simulink model "Microgrid_transition_model_FORFIG"  (R2020a)
settings: Solver=VariableStepAuto  StartTime=0.0  StopTime=16  MaxStep=1e-4  RelTol=1e-3
PreLoadFcn:
  | %run('FC_microgrid_param.m')
  | %load('gen_grid_init.mat')
InitFcn:
  | %load myisoModel_init;
  | run('FC_microgrid_param.m')
  | tic
  | run('CARTinitFcn.m')
  | %caseNo = 2;
  | 
  | %if (caseNo == 1)
  | %set_param(['Isolated_grid_paper_model_022521/SignalGen'], 'ActiveScenario', 'PStep222kW');
  | %else
  | %set_param(['Isolated_grid_paper_model_022521/SignalGen'], 'ActiveScenario', 'QStep222kVAr');
  | 
  | %end;
StopFcn:
  | toc
undefined symbols (not defined in the file): breakpoints1, breakpoints2, cp_table_data, ctrl, D1, Delta, DiscIntNeverNeededParam, DT, FC_BESS, find_system, gcbh, libFC_BESS, LowerLimit, magnitude, oversize, pq_ts, sps_rtmsupport, timer, Ts, ts, Ts_APC, Ts_Control, Ts_Power, UpperLimit
libraries: powerlib x130, powerlib_meascontrol x104, simulink x65, powerlib_extras x40, simulink_extras x16, eePowerMeasurement x9, sps_avr x7, pi_ctrl x4, spsDieselMotorModel x3, SignalEditorBlockLib x2, libLgBattery x1, libFC_PV x1
(part 5 of 13)

== system Microgrid_transition_model_FORFIG/Grid Feeder Protective Relay/RMS_Calculator2 ==
  note: % Copyright (c) 2016 Massachusetts Institute of Technology
      | % Permission is hereby granted, free of charge, to any person obtaining a copy of this
      | % software and associated documentation files (the "Software"), to deal in the Software
      | % without restriction, including without limitation the rights to use, copy, modify,
      | % merge, publish, distribute, sublicense, and/or sell copies of the Software, and to
      | % permit persons to whom the Software is furnished to do so, subject to the following
      | % conditions:
      | %
      | %
      | % The above copyright notice and this permission notice shall be included in
      | % all copies or substantial portions of the Software.
      | %
      | % THE SOFTWARE IS PROVIDED "AS IS", WITHOUT WARRANTY OF ANY KIND, EXPRESS OR IMPLIED,
      | % INCLUDING BUT NOT LIMITED TO THE WARRANTIES OF MERCHANTABILITY, FITNESS FOR A
      | % PARTICULAR PURPOSE AND NONINFRINGEMENT. IN NO EVENT SHALL THE AUTHORS OR COPYRIGHT
      | % HOLDERS BE LIABLE FOR ANY CLAIM, DAMAGES OR OTHER LIABILITY, WHETHER IN AN ACTION
      | % OF CONTRACT, TORT OR OTHERWISE, ARISING FROM, OUT OF OR IN CONNECTION WITH THE
      | % SOFTWARE OR THE USE OR OTHER DEALINGS IN THE SOFTWARE.
      | %
      | %
      | %%
  s : Inport
  Abs : Abs
  Discrete Mean value6 : powerlib_extras/Discrete Measurements/Discrete  Mean value  Freq=60  Vinit=0  Ts=Ts
      settings: SourceProductBaseCode=PS
  Product3 : Product  RndMeth=Zero
  Signed Sqrt : Sqrt  SaturateOnIntegerOverflow=on
  RMS : Outport
  wires:
  Signed Sqrt/1 -> RMS/1
  Discrete Mean value6/1 -> Abs/1
  s/1 -> Product3/2, Product3/1
  Product3/1 -> Discrete Mean value6/1
  Abs/1 -> Signed Sqrt/1

== system Microgrid_transition_model_FORFIG/Grid Feeder Protective Relay1/CS Modified PLL ==
  note: SPS Discrete 3-phase PLL
  note: Pierre Giroux, Gilbert Sybille
      | Power System Laboratory, IREQ
      | Hydro-Quebec
      | (August 2007)
  Vabc(pu) : Inport  PortDimensions=3
  2nd-Order Filter : powerlib_extras/Discrete  Control Blocks/Discrete  2nd-Order Filter  FilterType=Lowpass  Fo=25  Zeta=0.707  Ts=Ts  Initialize=on  Vac_Init=[0 0 Finit]  Vdc_Init=Finit  PlotResponse=off  param1=[1 500 0.1]
      settings: SourceProductBaseCode=PS
  Controller : Subsystem  mask(Discrete PID Controller){Kp=Kp, Ki=Ki, Kd=Kd, Par_Limits=[Flim(2) Flim(1)]*2*pi, Init=2*pi*Finit, Ts=Ts}
      mask prompts: Kp "Proportional gain (Kp):"; Ki "Integral gain (Ki):"; Kd "Derivative gain (Kd):"; Par_Limits "Output limits: [ Upper   Lower ]"; Init "Output initial value:"; Ts "Sample time:"
      mask help: This block implements a discrete PID controller.
      mask init:
      | UpperLimit=Par_Limits(1);
      | LowerLimit=Par_Limits(2);
      | power_initmask();
      settings: OpenFcn=power_openblockproxy();
      mask Display: disp('PID');
  Discrete Rate Limiter : powerlib_extras/Discrete  Control Blocks/Discrete Rate Limiter  R=12  F=-12  Vinit=Finit  Ts=Ts
      settings: SourceProductBaseCode=PS
  Discrete Mean value : powerlib_extras/Discrete Measurements/Discrete  Mean value  Freq=60  Vinit=0  Ts=Ts
      settings: SourceProductBaseCode=PS
  Gain10 : Gain  Gain=1/2/pi  SaturateOnIntegerOverflow=on  OutDataTypeStr=Inherit: Same as input  ParamDataTypeStr=Inherit: Same as input
  Mux2 : Mux  Inputs=2
  Selector : Selector  InputPortWidth=3  IndexOptions=Index vector (dialog)  Indices=2  OutputSizes=1
  Trigonometric Function : Trigonometry
  Trigonometric Function2 : Trigonometry  Operator=cos
  Unit Delay : UnitDelay  InitialCondition=Finit  SampleTime=Ts  HasFrameUpgradeWarning=on
  VCO : Subsystem
  abc_to_dq0 Transformation : powerlib_extras/Measurements/abc_to_dq0 Transformation
      settings: SourceProductBaseCode=PS
  Freq : Outport
  wt : Outport  Port=2
  Sin_Cos : Outport  Port=3
  wires:
  Discrete Mean value/1 -> Controller/1(Error)
  Controller/1(Out) -> VCO/1(w), Gain10/1  "W"
  Vabc(pu)/1 -> abc_to_dq0 Transformation/1
  abc_to_dq0 Transformation/1 -> Selector/1
  VCO/1(theta) -> Trigonometric Function/1, Trigonometric Function2/1, wt/1
  Trigonometric Function/1 -> Mux2/1
  Trigonometric Function2/1 -> Mux2/2
  Mux2/1 -> abc_to_dq0 Transformation/2, Sin_Cos/1
  Gain10/1 -> Discrete Rate Limiter/1
  Discrete Rate Limiter/1 -> 2nd-Order Filter/1
  Unit Delay/1 -> Freq/1
  2nd-Order Filter/1 -> Unit Delay/1
  Selector/1 -> Discrete Mean value/1  "Vq"

== system Microgrid_transition_model_FORFIG/Grid Feeder Protective Relay1/CS Modified PLL1 ==
  note: SPS Discrete 3-phase PLL
  note: Pierre Giroux, Gilbert Sybille
      | Power System Laboratory, IREQ
      | Hydro-Quebec
      | (August 2007)
  Vabc(pu) : Inport  PortDimensions=3
  2nd-Order Filter : powerlib_extras/Discrete  Control Blocks/Discrete  2nd-Order Filter  FilterType=Lowpass  Fo=25  Zeta=0.707  Ts=Ts  Initialize=on  Vac_Init=[0 0 Finit]  Vdc_Init=Finit  PlotResponse=off  param1=[1 500 0.1]
      settings: SourceProductBaseCode=PS
  Controller : Subsystem  mask(Discrete PID Controller){Kp=Kp, Ki=Ki, Kd=Kd, Par_Limits=[Flim(2) Flim(1)]*2*pi, Init=2*pi*Finit, Ts=Ts}
      mask prompts: Kp "Proportional gain (Kp):"; Ki "Integral gain (Ki):"; Kd "Derivative gain (Kd):"; Par_Limits "Output limits: [ Upper   Lower ]"; Init "Output initial value:"; Ts "Sample time:"
      mask help: This block implements a discrete PID controller.
      mask init:
      | UpperLimit=Par_Limits(1);
      | LowerLimit=Par_Limits(2);
      | power_initmask();
      settings: OpenFcn=power_openblockproxy();
      mask Display: disp('PID');
  Discrete Rate Limiter : powerlib_extras/Discrete  Control Blocks/Discrete Rate Limiter  R=12  F=-12  Vinit=Finit  Ts=Ts
      settings: SourceProductBaseCode=PS
  Discrete Mean value : powerlib_extras/Discrete Measurements/Discrete  Mean value  Freq=60  Vinit=0  Ts=Ts
      settings: SourceProductBaseCode=PS
  Gain10 : Gain  Gain=1/2/pi  SaturateOnIntegerOverflow=on  OutDataTypeStr=Inherit: Same as input  ParamDataTypeStr=Inherit: Same as input
  Mux2 : Mux  Inputs=2
  Selector : Selector  InputPortWidth=3  IndexOptions=Index vector (dialog)  Indices=2  OutputSizes=1
  Trigonometric Function : Trigonometry
  Trigonometric Function2 : Trigonometry  Operator=cos
  Unit Delay : UnitDelay  InitialCondition=Finit  SampleTime=Ts  HasFrameUpgradeWarning=on
  VCO : Subsystem
  abc_to_dq0 Transformation : powerlib_extras/Measurements/abc_to_dq0 Transformation
      settings: SourceProductBaseCode=PS
  Freq : Outport
  wt : Outport  Port=2
  Sin_Cos : Outport  Port=3
  wires:
  Discrete Mean value/1 -> Controller/1(Error)
  Controller/1(Out) -> VCO/1(w), Gain10/1  "W"
  Vabc(pu)/1 -> abc_to_dq0 Transformation/1
  abc_to_dq0 Transformation/1 -> Selector/1
  VCO/1(theta) -> Trigonometric Function/1, Trigonometric Function2/1, wt/1
  Trigonometric Function/1 -> Mux2/1
  Trigonometric Function2/1 -> Mux2/2
  Mux2/1 -> abc_to_dq0 Transformation/2, Sin_Cos/1
  Gain10/1 -> Discrete Rate Limiter/1
  Discrete Rate Limiter/1 -> 2nd-Order Filter/1
  Unit Delay/1 -> Freq/1
  2nd-Order Filter/1 -> Unit Delay/1
  Selector/1 -> Discrete Mean value/1  "Vq"

== system Microgrid_transition_model_FORFIG/Grid Feeder Protective Relay1/R25 - Sync Check v0.1 ==
  note: Copyright 2018 Alliance for Sustainable Energy, LLC
      |
      | Permission is hereby granted, free of charge, to any person obtaining a copy of this software
      | and associated documentation files (the "Software"), to deal in the Software without restriction,
      | including without limitation the rights to use, copy, modify, merge, publish, distribute, sublicense,
      | and/or sell copies of the Software, and to permit persons to whom the Software is furnished to do so,
      | subject to the following conditions:
      |
      | The above copyright notice and this permission notice shall be included in all copies or substantial portions of the Software.
      |
      | THE SOFTWARE IS PROVIDED "AS IS", WITHOUT WARRANTY OF ANY KIND, EXPRESS OR IMPLIED, INCLUDING
      | BUT NOT LIMITED TO THE WARRANTIES OF MERCHANTABILITY, FITNESS FOR A PARTICULAR PURPOSE AND
      | NONINFRINGEMENT. IN NO EVENT SHALL THE AUTHORS, THE COPYRIGHT HOLDERS, THE UNITED STATES,
      | THE UNITED STATES DEPARTMENT OF ENERGY, OR ANY OF THEIR EMPLOYEES BE LIABLE FOR ANY CLAIM,
      | DAMAGES OR OTHER LIABILITY, WHETHER IN AN ACTION OF CONTRACT, TORT OR OTHERWISE, ARISING FROM,
      | OUT OF OR IN CONNECTION WITH THE SOFTWARE OR THE USE OR OTHER DEALINGS IN THE SOFTWARE.
  note: true: If the life bus has voltage > 0.9pu and the other bus has voltage < threshold
      | true: both sides of the breaker are deadbuses
  note: voltage difference
  note: frequency difference
  note: angle difference
  note: * this block checks for synchronism based on phase A only
      | * the block also implements a deadbus logic
  VPKLN_bus : Inport
  VPKLN_line : Inport  Port=2
  pll_data : Inport  Port=3
  relay_param : Inport  Port=4
  Bus Creator : BusCreator  Inputs=3
  Bus Selector : BusSelector  OutputSignals=VRMSLL,dV_threshold,angle_threshold,dF_threshold
  Bus Selector1 : BusSelector  OutputSignals=freq_bus,freq_line,wt_bus,wt_line
  Demux : Demux  Outputs=3
  Demux1 : Demux  Outputs=3
  Demux10 : Demux  Outputs=2
  Freq_Comparator : Subsystem
  Logical Operator : Logic  Inputs=3  AllPortsSameDT=off  OutDataTypeStr=boolean
  Logical Operator3 : Logic  Operator=OR  AllPortsSameDT=off  OutDataTypeStr=boolean
  Mux1 : Mux  Inputs=2
  Phase_Comparator : Subsystem
  Scope{,1..3} (4 alike) : Scope  NumInputPorts=3
  Terminator{5..8} (4 alike) : Terminator
  Voltage_Comparator : Subsystem
  deadbus fcn : MATLAB Function  TreatAsAtomicUnit=on
  dMeas : Outport
  R25 : Outport  Port=2
  wires:
  Logical Operator3/1 -> R25/1
  pll_data/1 -> Bus Selector1/1
  Logical Operator/1 -> Logical Operator3/2  "dV&dF&dW"
  deadbus fcn/1(y) -> Logical Operator3/1  "deadbus"
  VPKLN_line/1 -> Demux1/1
  VPKLN_bus/1 -> Demux/1
  Demux/3 -> Terminator8/1
  Demux/2 -> Terminator7/1
  Demux1/3 -> Terminator5/1
  Demux1/2 -> Terminator6/1
  Demux1/1 -> Mux1/2
  Demux/1 -> Mux1/1  "a_sys"
  Mux1/1 -> Demux10/1  "RMSLL"
  relay_param/1 -> Bus Selector/1
  Bus Selector/1 -> [VRMSLL]  "<VRMSLL>"
  Bus Selector/2 -> [dV_threshold]  "<dV_threshold>"
  Bus Selector/3 -> [angle_threshold]  "<angle_threshold>"
  Bus Selector/4 -> [dF_threshold]  "<dF_threshold>"
  Voltage_Comparator/2(dV) -> Bus Creator/3  "dV"
  Freq_Comparator/2(dF) -> Bus Creator/2  "dF"
  Phase_Comparator/2(dWt) -> Bus Creator/1  "dWt"
  Bus Creator/1 -> dMeas/1
  Freq_Comparator/1(Locked) -> Scope/2, Logical Operator/2  "dF"
  Voltage_Comparator/1(Locked) -> Scope/1, Logical Operator/1  "dV"
  Phase_Comparator/1(Locked) -> Scope/3, Logical Operator/3  "dW"
  [dV_threshold] -> Voltage_Comparator/3(dV_threshold), Scope1/3
  Demux10/1 -> Scope1/1, Voltage_Comparator/1(V_bus), deadbus fcn/1(Vbus)  "vbus"
  Demux10/2 -> Scope1/2, Voltage_Comparator/2(V_line), deadbus fcn/2(Vline)  "vline"
  Bus Selector1/1 -> Scope2/1, Freq_Comparator/1(f_grid)  "<freq_bus>"
  Bus Selector1/2 -> Scope2/2, Freq_Comparator/2(f_gen)  "<freq_line>"
  [dF_threshold] -> Scope2/3, Freq_Comparator/3(dF_threshold)
  [angle_threshold] -> Scope3/3, Phase_Comparator/3(angle_threshold)
  Bus Selector1/4 -> Scope3/2, Phase_Comparator/2(wt_gen)  "<wt_line>"
  Bus Selector1/3 -> Scope3/1, Phase_Comparator/1(wt_grid)  "<wt_bus>"

== system Microgrid_transition_model_FORFIG/Grid Feeder Protective Relay1/RMS_Calculator1 ==
  note: % Copyright (c) 2016 Massachusetts Institute of Technology
      | % Permission is hereby granted, free of charge, to any person obtaining a copy of this
      | % software and associated documentation files (the "Software"), to deal in the Software
      | % without restriction, including without limitation the rights to use, copy, modify,
      | % merge, publish, distribute, sublicense, and/or sell copies of the Software, and to
      | % permit persons to whom the Software is furnished to do so, subject to the following
      | % conditions:
      | %
      | %
      | % The above copyright notice and this permission notice shall be included in
      | % all copies or substantial portions of the Software.
      | %
      | % THE SOFTWARE IS PROVIDED "AS IS", WITHOUT WARRANTY OF ANY KIND, EXPRESS OR IMPLIED,
      | % INCLUDING BUT NOT LIMITED TO THE WARRANTIES OF MERCHANTABILITY, FITNESS FOR A
      | % PARTICULAR PURPOSE AND NONINFRINGEMENT. IN NO EVENT SHALL THE AUTHORS OR COPYRIGHT
      | % HOLDERS BE LIABLE FOR ANY CLAIM, DAMAGES OR OTHER LIABILITY, WHETHER IN AN ACTION
      | % OF CONTRACT, TORT OR OTHERWISE, ARISING FROM, OUT OF OR IN CONNECTION WITH THE
      | % SOFTWARE OR THE USE OR OTHER DEALINGS IN THE SOFTWARE.
      | %
      | %
      | %%
  s : Inport
  Abs : Abs
  Discrete Mean value6 : powerlib_extras/Discrete Measurements/Discrete  Mean value  Freq=60  Vinit=0  Ts=Ts
      settings: SourceProductBaseCode=PS
  Product3 : Product  RndMeth=Zero
  Signed Sqrt : Sqrt  SaturateOnIntegerOverflow=on
  RMS : Outport
  wires:
  Abs/1 -> Signed Sqrt/1
  Product3/1 -> Discrete Mean value6/1
  s/1 -> Product3/1, Product3/2
  Discrete Mean value6/1 -> Abs/1
  Signed Sqrt/1 -> RMS/1

== system Microgrid_transition_model_FORFIG/Grid Feeder Protective Relay1/RMS_Calculator2 ==
  note: % Copyright (c) 2016 Massachusetts Institute of Technology
      | % Permission is hereby granted, free of charge, to any person obtaining a copy of this
      | % software and associated documentation files (the "Software"), to deal in the Software
      | % without restriction, including without limitation the rights to use, copy, modify,
      | % merge, publish, distribute, sublicense, and/or sell copies of the Software, and to
      | % permit persons to whom the Software is furnished to do so, subject to the following
      | % conditions:
      | %
      | %
      | % The above copyright notice and this permission notice shall be included in
      | % all copies or substantial portions of the Software.
      | %
      | % THE SOFTWARE IS PROVIDED "AS IS", WITHOUT WARRANTY OF ANY KIND, EXPRESS OR IMPLIED,
      | % INCLUDING BUT NOT LIMITED TO THE WARRANTIES OF MERCHANTABILITY, FITNESS FOR A
      | % PARTICULAR PURPOSE AND NONINFRINGEMENT. IN NO EVENT SHALL THE AUTHORS OR COPYRIGHT
      | % HOLDERS BE LIABLE FOR ANY CLAIM, DAMAGES OR OTHER LIABILITY, WHETHER IN AN ACTION
      | % OF CONTRACT, TORT OR OTHERWISE, ARISING FROM, OUT OF OR IN CONNECTION WITH THE
      | % SOFTWARE OR THE USE OR OTHER DEALINGS IN THE SOFTWARE.
      | %
      | %
      | %%
  s : Inport
  Abs : Abs
  Discrete Mean value6 : powerlib_extras/Discrete Measurements/Discrete  Mean value  Freq=60  Vinit=0  Ts=Ts
      settings: SourceProductBaseCode=PS
  Product3 : Product  RndMeth=Zero
  Signed Sqrt : Sqrt  SaturateOnIntegerOverflow=on
  RMS : Outport
  wires:
  Abs/1 -> Signed Sqrt/1
  Product3/1 -> Discrete Mean value6/1
  s/1 -> Product3/1, Product3/2
  Discrete Mean value6/1 -> Abs/1
  Signed Sqrt/1 -> RMS/1

== system Microgrid_transition_model_FORFIG/Microgrid controller/ResyncControl ==
  note: Shorcut fix for frequency offset?
      | Secondary freq control?
  ProtRelayMeas : Inport
  <StartResync> : Inport  Port=2
  AND : Logic  IconShape=distinctive  AllPortsSameDT=off  OutDataTypeStr=boolean
  Add : Sum
  Bus Selector : BusSelector  OutputSignals=R25_Meas.dWt,R25_Meas.dF,Closed,R25_Meas.dV
  Constant : Constant  Value=0.0/60
  Discrete-Time Integrator : DiscreteIntegrator  ExternalReset=level  InitialCondition=1  SampleTime=Ts  ICPrevOutput=DiscIntNeverNeededParam  ICPrevScaledInput=DiscIntNeverNeededParam
  Discrete-Time Integrator1 : DiscreteIntegrator  ExternalReset=level  InitialCondition=1  SampleTime=Ts  ICPrevOutput=DiscIntNeverNeededParam  ICPrevScaledInput=DiscIntNeverNeededParam
  Gain : Gain  Gain=-0.05
  Gain1 : Gain  Gain=-5
  Gain2 : Gain  Gain=0.5
  NOT : Logic  Operator=NOT  IconShape=distinctive  AllPortsSameDT=off  OutDataTypeStr=boolean
  NOT1 : Logic  Operator=NOT  IconShape=distinctive  AllPortsSameDT=off  OutDataTypeStr=boolean
  Sum : Sum  Inputs=|++
  f_ref : Outport
  v_ref : Outport  Port=2
  wires:
  ProtRelayMeas/1 -> Bus Selector/1
  Gain/1 -> Discrete-Time Integrator/1
  NOT/1 -> AND/1
  Bus Selector/3 -> NOT/1  "<Closed>"
  Gain1/1 -> Discrete-Time Integrator1/1
  AND/1 -> NOT1/1
  Bus Selector/1 -> Gain2/1  "<dWt>"
  Gain2/1 -> Add/1
  Bus Selector/4 -> Gain1/1  "<dV>"
  NOT1/1 -> Discrete-Time Integrator/2, Discrete-Time Integrator1/2
  <StartResync>/1 -> AND/2
  Add/1 -> Gain/1
  Discrete-Time Integrator1/1 -> v_ref/1  "v_ref"
  Bus Selector/2 -> Add/2  "<dF>"
  Discrete-Time Integrator/1 -> Sum/1  "f_ref"
  Sum/1 -> f_ref/1  "f_ref"
  Constant/1 -> Sum/2

== system Microgrid_transition_model_FORFIG/Subsystem4/Generator Bus ==
  Grid Bus1 : powerlib/Measurements/Three-Phase V-I Measurement  VoltageMeasurement=phase-to-ground  SetLabelV=on  LabelV=Vwind  Vpu=off  VpuLL=off  CurrentMeasurement=yes  SetLabelI=on  LabelI=Iwind  Ipu=off  Pbase=100e6  Vbase=(25000)*1.00007  OutputType=Complex  PhasorSimulation=off  PSBequivalent=0
  A : PMIOPort  Side=Left
  a : PMIOPort  Port=2  Side=Right
  B : PMIOPort  Port=3  Side=Left
  b : PMIOPort  Port=4  Side=Right
  C : PMIOPort  Port=5  Side=Left
  c : PMIOPort  Port=6  Side=Right
  connections:
  Grid Bus1/RConn1 -- a/RConn1
  Grid Bus1/RConn2 -- b/RConn1
  Grid Bus1/RConn3 -- c/RConn1
  C/RConn1 -- Grid Bus1/LConn3
  B/RConn1 -- Grid Bus1/LConn2
  A/RConn1 -- Grid Bus1/LConn1

== system Microgrid_transition_model_FORFIG/Wind Turbine Type 4/APC (atomic)1 ==
  note: Cases
      | 1 IR
      | 2 PFR
      | 3 P/Q
      | 4 Vrms
      | 5 Baseline
  Freq (Hz) : Inport
  wr [pu] : Inport  Port=2
  Pin : Inport  Port=3
  case : Inport  Port=4
  Qin : Inport  Port=5
  protection : Inport  Port=6
  Baseline : Subsystem
  Constant : Constant
  Constant1 : Constant
  Constant2 : Constant  Value=0
  Constant3 : Constant
  Constant4 : Constant  Value=0.8
  Divide : Product  Inputs=**
  Divide1 : Product  Inputs=**
  Divide2 : Product  Inputs=**
  From Spreadsheet : FromSpreadsheet  FileName=cmd_timeseries.xlsx  SheetName=T  SampleTime=0.01
  Inertial Response (to df) : Subsystem
  Manual Switch : ManualSwitch  CurrentSetting=0
  Merge : Merge  Inputs=5
  Merge1 : Merge  Inputs=5
  Merge2 : Merge  Inputs=5
  PFR : Subsystem
  PQ : Subsystem
  Saturation1 : Saturate  UpperLimit=1  LowerLimit=0
  Scope : Scope  NumInputPorts=2
  Scope1 : Scope  NumInputPorts=2
  Sum : Sum  Inputs=|++
  Sum1 : Sum  Inputs=|++
  Switch Case : SwitchCase  CaseConditions={1,2,3,4,5}
  Switch1 : Switch  Criteria=u2 > Threshold
  Switch2 : Switch  Criteria=u2 > Threshold  Threshold=1
  VR (handled by FRT) : Subsystem
  When to start PFR/SFR : DigitalClock  SampleTime=-1
  When to start PFR/SFR1 : DigitalClock  SampleTime=-1
  Pcmd : Outport
  Tcmd : Outport  Port=2
  Qcmd : Outport  Port=3
  wires:
  Sum/1 -> Manual Switch/2
  From Spreadsheet/1 -> Manual Switch/1  "Tgain"
  Saturation1/1 -> Scope/2, Divide1/1
  Switch2/1 -> Divide2/1
  protection/1 -> Divide/2, Scope/1, Divide1/2, Divide2/2
  Divide/1 -> Scope1/2, Tcmd/1
  Divide2/1 -> Qcmd/1
  Merge1/1 -> Switch2/1
  Constant2/1 -> Switch2/3
  When to start PFR/SFR1/1 -> Switch2/2
  VR (handled by FRT)/3(dT) -> Merge/4
  VR (handled by FRT)/2(dP) -> Merge2/4
  PQ/3(dT) -> Merge2/3
  PFR/3(Qcmd) -> Merge1/2
  PFR/2(dT) -> Merge2/2
  Inertial Response (to df)/3(Qcmd) -> Merge1/1
  Inertial Response (to df)/2(dP) -> Merge/1
  PQ/1(dP) -> Merge/3
  Switch Case/3 -> PQ/Action
  Switch Case/4 -> VR (handled by FRT)/Action
  case/1 -> Switch Case/1
  wr [pu]/1 -> Inertial Response (to df)/3(wg (pu))
  Switch Case/1 -> Inertial Response (to df)/Action
  Qin/1 -> PQ/2(Qin)
  Constant3/1 -> Sum1/2
  Switch Case/2 -> PFR/Action
  Pin/1 -> PQ/1(SFRcmd)
  Constant1/1 -> Sum/2
  PFR/1(dP) -> Merge/2
  Freq (Hz)/1 -> Inertial Response (to df)/1(Freq (Hz)), PFR/1(Freq (Hz))
  VR (handled by FRT)/1(Qcmd) -> Merge1/4
  Sum1/1 -> Switch1/1
  Baseline/1(Qcmd) -> Merge1/5
  Merge/1 -> Sum1/1
  Switch Case/5 -> Baseline/Action
  Constant4/1 -> Switch1/3
  Merge2/1 -> Sum/1
  PQ/2(Qcmd) -> Merge1/3
  Baseline/3(dT) -> Merge2/5
  When to start PFR/SFR/1 -> Switch1/2
  Constant/1 -> Inertial Response (to df)/2(type1)
  Switch1/1 -> Saturation1/1
  Manual Switch/1 -> Scope1/1, Divide/1
  Inertial Response (to df)/1(dT) -> Merge2/1
  Divide1/1 -> Pcmd/1
  Baseline/2(dP) -> Merge/5

== system Microgrid_transition_model_FORFIG/Wind Turbine Type 4/Average Switch Voltage ==
  Vswitch : Inport
  Diode : powerlib/Power Electronics/Diode  Ron=1e-6/Nb_wt  Lon=0  Vf=0  IC=0  UseSnubber=off  Rs=1e5  Cs=inf  Measurements=off
      settings: SourceProductBaseCode=MT,PS
  V : powerlib/Electrical Sources/Controlled Voltage Source  Initialize=on  Source_Type=AC  Amplitude=0  Phase=0  Frequency=0  Measurements=None
      settings: SourceProductBaseCode=MT,PS
  + : PMIOPort  Side=Right
  - : PMIOPort  Port=2  Side=Left
  wires:
  Vswitch/1 -> V/1
  connections:
  Diode/RConn1 -- V/RConn1
  +/RConn1 -- Diode/LConn1
  -/RConn1 -- V/LConn1

== system Microgrid_transition_model_FORFIG/Wind Turbine Type 4/Control ==
  note: Inputs
  note: Grid-Side Converter
      | Control System
  note: Speed Regulator & Pitch Control
  note: Excitation
      | Control system
  Vabc_grid : Inport
  Iabc_grid_conv : Inport  Port=2
  Vabc_LL_stator : Inport  Port=3
  Iabc_stator : Inport  Port=4
  IL : Inport  Port=5
  Vdc : Inport  Port=6
  angle_rotor : Inport  Port=7
  wr : Inport  Port=8
  Qref : Inport  Port=9
  Pcmd : Inport  Port=10
  Tgain : Inport  Port=11
  AS mode : Inport  Port=12
  Bus Creator : BusCreator  Inputs=2
  Excitation Control system : Subsystem
  Grid-Side Inverter Control : Subsystem
  Measurement and Transformation : Subsystem
  Speed & Pitch Control1 : Subsystem
  Unit Delay : UnitDelay  SampleTime=-1  HasFrameUpgradeWarning=on
  Unit Delay{2,5..8} (5 alike) : UnitDelay  SampleTime=Ts  HasFrameUpgradeWarning=on
  U_ctrl_inverter : Outport
  Duty_Cycle : Outport  Port=2  VectorParamsAs1DForOutWhenUnconnected=off
  Pitch_angle : Outport  Port=3  VectorParamsAs1DForOutWhenUnconnected=off
  Vf : Outport  Port=4  VectorParamsAs1DForOutWhenUnconnected=off
  PQ_pu : Outport  Port=5  VectorParamsAs1DForOutWhenUnconnected=off
  protection : Outport  Port=6
  tag scope: Idq_gc=global, Theta_PLL=global, Vdc_meas=global, Vdq_grid=global, Vmeas=global, w_pu=global
  wires:
  Excitation Control system/1(Vf) -> Unit Delay2/1
  Measurement and Transformation/7(Qmeas) -> [Qmeas]
  Measurement and Transformation/1(Vdq_grid) -> [Vdq_grid]
  Measurement and Transformation/2(Idq_gc) -> [Idq_gc]
  Measurement and Transformation/6(Pmeas) -> [Pmeas]
  Measurement and Transformation/8(Vmeas) -> [Vmeas]
  Measurement and Transformation/10(w_pu) -> [w_pu]
  Measurement and Transformation/5(Vdc_meas) -> [Vdc_meas]
  Measurement and Transformation/11("wr ") -> [wr]
  Measurement and Transformation/12("Qref ") -> [Qref]
  Measurement and Transformation/4(Flux) -> [Flux]
  [Flux] -> Excitation Control system/1(Flux)
  [wr] -> Excitation Control system/2(wr)
  Vabc_grid/1 -> Measurement and Transformation/1(Vabc_grid)
  Iabc_grid_conv/1 -> Measurement and Transformation/2(Iabc_gc)
  Vabc_LL_stator/1 -> Measurement and Transformation/3(Vabc_LL_s)
  Iabc_stator/1 -> Measurement and Transformation/4(Iabc_s)
  Vdc/1 -> Measurement and Transformation/6(Vdc)
  Qref/1 -> Measurement and Transformation/7(Qref)
  angle_rotor/1 -> Measurement and Transformation/8(angle_rotor)
  wr/1 -> Measurement and Transformation/9(wr)
  Measurement and Transformation/9(Theta_PLL) -> [Theta_PLL]
  Bus Creator/1 -> [PQ_pu], PQ_pu/1
  Unit Delay2/1 -> Vf/1
  [Pmeas] -> Unit Delay6/1
  [Qmeas] -> Unit Delay7/1
  Unit Delay6/1 -> Bus Creator/1  "P_pu"
  Unit Delay7/1 -> Bus Creator/2  "Q_pu"
  Measurement and Transformation/3("IL ") -> [IL]
  IL/1 -> Measurement and Transformation/5(IL)
  Grid-Side Inverter Control/2(Uctrl_inverter) -> Unit Delay/1
  [PQ_pu] -> Grid-Side Inverter Control/2(PQ_meas)
  Grid-Side Inverter Control/1(protection) -> protection/1
  [u_f_protect] -> Grid-Side Inverter Control/5(u_f_protect)
  Unit Delay/1 -> U_ctrl_inverter/1
  [u_frt] -> Grid-Side Inverter Control/4(u_frt)
  [w_pu] -> Grid-Side Inverter Control/7(w_pu)
  [Qref] -> Grid-Side Inverter Control/1(Q_ref)
  [Idq_gc] -> Grid-Side Inverter Control/6(Idq_gc)
  [Vdq_grid] -> Grid-Side Inverter Control/8(Vdq_grid)
  [Vdc_meas] -> Grid-Side Inverter Control/3(Vdc_meas)
  [Theta_PLL] -> Grid-Side Inverter Control/9(Theta_PLL)
  Measurement and Transformation/13(u_frt) -> [u_frt]
  Measurement and Transformation/14(u_f_protect) -> [u_f_protect]
  Tgain/1 -> Speed & Pitch Control1/4(Tgain)
  [wr] -> Speed & Pitch Control1/1(wr)
  [IL] -> Speed & Pitch Control1/3(IL)
  Speed & Pitch Control1/1(Duty_Cycle) -> Unit Delay5/1
  [Pmeas] -> Speed & Pitch Control1/2(Pmeas)
  Speed & Pitch Control1/2(Pitch (deg)) -> Unit Delay8/1
  Pcmd/1 -> Speed & Pitch Control1/5(Pref)
  Unit Delay5/1 -> Duty_Cycle/1
  Unit Delay8/1 -> Pitch_angle/1
  AS mode/1 -> Grid-Side Inverter Control/10(AS mode)

== system Microgrid_transition_model_FORFIG/Wind Turbine Type 4/Drive Train ==
  note: Shaft
  note: Turbine
  note: Wind turbine drive train based on a 2-masse model
  T_wt (pu) : Inport
  Generator speed (pu) : Inport  Port=2
  1_2H_WT : Gain  Gain=1/(2*H_WT)  SaturateOnIntegerOverflow=on  OutDataTypeStr=Inherit: Same as input  ParamDataTypeStr=Inherit: Same as input
  Discrete-Time Integrator : DiscreteIntegrator  InitialCondition=w_wt0  SampleTime=Ts  ICPrevOutput=DiscIntNeverNeededParam  ICPrevScaledInput=DiscIntNeverNeededParam
  Discrete-Time Integrator1 : DiscreteIntegrator  InitialCondition=torque0/Ksh  SampleTime=Ts  ICPrevOutput=DiscIntNeverNeededParam  ICPrevScaledInput=DiscIntNeverNeededParam
  Mutual damping : Gain  Gain=D_mutual  SaturateOnIntegerOverflow=on  OutDataTypeStr=Inherit: Same as input  ParamDataTypeStr=Inherit: Same as input
  Stiffness : Gain  Gain=Ksh  SaturateOnIntegerOverflow=on  OutDataTypeStr=Inherit: Same as input  ParamDataTypeStr=Inherit: Same as input
  Sum : Sum  Inputs=+-  InputSameDT=on  SaturateOnIntegerOverflow=on  OutDataTypeStr=Inherit: Same as first input
  Sum1 : Sum  Inputs=+-  InputSameDT=on  SaturateOnIntegerOverflow=on  OutDataTypeStr=Inherit: Same as first input
  Sum2 : Sum  InputSameDT=on  SaturateOnIntegerOverflow=on  OutDataTypeStr=Inherit: Same as first input
  wbase : Gain  Gain=wbase  SaturateOnIntegerOverflow=on  OutDataTypeStr=Inherit: Same as input  ParamDataTypeStr=Inherit: Same as input
  W_wt (pu) : Outport  VectorParamsAs1DForOutWhenUnconnected=off
  T_shaft (pu) : Outport  Port=2  VectorParamsAs1DForOutWhenUnconnected=off
  wires:
  wbase/1 -> Discrete-Time Integrator1/1
  Discrete-Time Integrator1/1 -> Stiffness/1
  Stiffness/1 -> Sum2/1
  Sum/1 -> 1_2H_WT/1
  1_2H_WT/1 -> Discrete-Time Integrator/1
  Discrete-Time Integrator/1 -> Sum1/1, W_wt (pu)/1
  Generator speed (pu)/1 -> Sum1/2
  Sum1/1 -> wbase/1, Mutual damping/1
  Mutual damping/1 -> Sum2/2
  Sum2/1 -> Sum/2, T_shaft (pu)/1
  T_wt (pu)/1 -> Sum/1

== system Microgrid_transition_model_FORFIG/Wind Turbine Type 4/Fault Controller (atomic)  ==
  Inport : Inport
  1-s avg : powerlib_meascontrol/Measurements/Mean  Freq=1  Vinit=0  Ts=Ts_APC
  Bus Creator : BusCreator  Inputs=4
  Bus Selector : BusSelector  OutputSignals=T,modeValue,Tfuture
  Bus Selector2 : BusSelector  OutputSignals=TRP,TNA,TS
  Constant : Constant  Value=0.01
  Delay : Delay  DelayLength=1  InitialCondition=ctrl
  Delay1 : Delay  DelayLength=1  InitialCondition=timer
  From Spreadsheet1 : FromSpreadsheet  FileName=fault_timeseries.xlsx  SheetName=dT  SampleTime=-1
  From Spreadsheet2 : FromSpreadsheet  Commented=on  FileName=fault_timeseries.xlsx  SheetName=ax  SampleTime=DT
  From Spreadsheet5 : FromSpreadsheet  FileName=fault_timeseries.xlsx  SheetName=genTemp  SampleTime=-1
  From Spreadsheet6 : FromSpreadsheet  FileName=fault_timeseries.xlsx  SheetName=dwHSS  SampleTime=-1
  Manual Switch1 : ManualSwitch
  Mux : Mux  Inputs=3
  P derate override : Constant
  "turbine_safety " : MATLAB Function  TreatAsAtomicUnit=on
  savgP : Outport
  genTemp : Outport  Port=2
  dwHSS : Outport  Port=3
  Pderate : Outport  Port=4
  mode : Outport  Port=5
  Timers : Outport  Port=6
  dTemp : Outport  Port=7
  Ppredict : Outport  Port=8
  wires:
  From Spreadsheet5/1 -> genTemp/1, Bus Creator/2  "genTemp"
  "turbine_safety "/1(ctrl) -> Delay/1
  Delay1/1 -> "turbine_safety "/3("timer "), Bus Selector2/1
  Delay/1 -> "turbine_safety "/1("ctrl "), Bus Selector/1
  "turbine_safety "/2(timer) -> Delay1/1
  From Spreadsheet6/1 -> Bus Creator/3, dwHSS/1  "dwHSS"
  Bus Creator/1 -> "turbine_safety "/2(data)
  P derate override/1 -> Manual Switch1/1
  Inport/1 -> 1-s avg/1  "power"
  Bus Selector/2 -> mode/1  "<modeValue>"
  Bus Selector2/1 -> Mux/1  "<TRP>"
  Mux/1 -> Timers/1
  Constant/1 -> "turbine_safety "/4(dt)
  Bus Selector2/2 -> Mux/2  "<TNA>"
  From Spreadsheet1/1 -> Bus Creator/4, dTemp/1  "dT"
  Bus Selector2/3 -> Mux/3  "<TS>"
  Bus Selector/3 -> Ppredict/1  "<Tfuture>"
  1-s avg/1 -> savgP/1, Bus Creator/1  "savgP"
  Manual Switch1/1 -> Pderate/1
  Bus Selector/1 -> Manual Switch1/2  "<T>"

== system Microgrid_transition_model_FORFIG/Wind Turbine Type 4/Inverter and DC-DC Converter Average Models ==
  note: Pac=Vab*Ia -Vbc*Ic
      | Pdc=Vdc*Idc
  note: Vab Vbc Inverter
      | Average Model
  note: DC-DC Converter
      | Average Model
  note: Inverter and DC-DC Boost Converter
      | Average Models
  note: Current of the boost converter diode
      | This diode is not illustrated in the average model
  IL : Inport
  Iabc_grid_conv : Inport  Port=2
  Uctrl_inverter : Inport  Port=3
  Duty_Cycle : Inport  Port=4
  0.1 : Gain  Gain=0.5
  0.2 : Gain  Gain=-1
  0.5 : Gain  Gain=0.5
  1/C : Gain  Gain=1/C_DClink
  Constant2 : Constant
  Demux : Demux  Outputs=3
  Demux2 : Demux  Outputs=3
  Discrete-Time Integrator : DiscreteIntegrator  InitialCondition=Vdc_nom  SampleTime=Ts  LimitOutput=on  LowerSaturationLimit=eps  ICPrevOutput=DiscIntNeverNeededParam  ICPrevScaledInput=DiscIntNeverNeededParam
  Product{1..4,6..7} (6 alike) : Product  RndMeth=Zero
  Product5 : Product  Inputs=*/  RndMeth=Zero
  Saturation Dynamic : simulink/Discontinuities/Saturation Dynamic  OutMin=[]  OutMax=[]  OutDataTypeStr=Inherit: Same as second input  OutDataType=sfix(16)  OutScaling=2^-10  DoSatur=off
  Saturation Dynamic1 : simulink/Discontinuities/Saturation Dynamic  OutMin=[]  OutMax=[]  OutDataTypeStr=Inherit: Same as second input  OutDataType=sfix(16)  OutScaling=2^-10  DoSatur=off
  Scope : Scope
  Subtract1 : Sum  Inputs=+-
  Subtract2 : Sum  Inputs=+-
  Subtract3 : Sum  Inputs=+-
  Subtract4 : Sum
  Sum : Sum  Inputs=|+-
  Terminator : Terminator
  pu->A : Gain  Gain=Pnom/(3*sqrt(2)/pi*Vnom_gen)  SaturateOnIntegerOverflow=on  OutDataTypeStr=Inherit: Same as input  ParamDataTypeStr=Inherit: Same as input
  "pu->A " : Gain  Gain=Pnom/sqrt(3)/Vnom*sqrt(2)  SaturateOnIntegerOverflow=on  OutDataTypeStr=Inherit: Same as input  ParamDataTypeStr=Inherit: Same as input
  Vab (V) : Outport  VectorParamsAs1DForOutWhenUnconnected=off
  Vbc (V) : Outport  Port=2  VectorParamsAs1DForOutWhenUnconnected=off
  Vswitch (V) : Outport  Port=3  VectorParamsAs1DForOutWhenUnconnected=off
  Vdc (V) : Outport  Port=4  VectorParamsAs1DForOutWhenUnconnected=off
  wires:
  Product1/1 -> Vswitch (V)/1
  Product2/1 -> Scope/1, [Idiode]
  [Vdc] -> Product1/1
  IL/1 -> pu->A/1
  Sum/1 -> Product2/1, Product1/2
  Constant2/1 -> Sum/1
  1/C/1 -> Discrete-Time Integrator/1
  Discrete-Time Integrator/1 -> Vdc (V)/1, Product5/2, [Vdc]
  Subtract4/1 -> 1/C/1
  Demux/1 -> Product3/2  "Ia"
  "pu->A "/1 -> Demux/1
  Demux/2 -> Terminator/1
  Iabc_grid_conv/1 -> "pu->A "/1
  Duty_Cycle/1 -> Sum/2
  Product4/1 -> Subtract2/2
  Product3/1 -> Subtract2/1
  Subtract2/1 -> Product5/1  "Pac"
  Demux/3 -> Product4/2  "Ic"
  [Vab] -> Product3/1
  [Vbc] -> Product4/1
  Product5/1 -> Subtract4/2  "Idc grid converter"
  [Vdc] -> 0.2/1, Saturation Dynamic1/1, Saturation Dynamic/1, Product6/2, Product7/2
  Subtract1/1 -> Product7/1
  Subtract3/1 -> Product6/1
  Product7/1 -> 0.1/1
  Product6/1 -> 0.5/1
  Demux2/3 -> Subtract1/2
  Demux2/2 -> Subtract3/2, Subtract1/1
  Demux2/1 -> Subtract3/1
  0.5/1 -> Saturation Dynamic/2  "Vab_avg"
  0.1/1 -> Saturation Dynamic1/2  "Vbc_avg"
  0.2/1 -> Saturation Dynamic/3, Saturation Dynamic1/3
  Uctrl_inverter/1 -> Demux2/1
  Saturation Dynamic/1 -> Vab (V)/1, [Vab]
  Saturation Dynamic1/1 -> Vbc (V)/1, [Vbc]
  [Idiode] -> Subtract4/1  "Idiode"
  pu->A/1 -> Product2/2

== system Microgrid_transition_model_FORFIG/Wind Turbine Type 4/Wind Turbine1 ==
  W_wt (pu) : Inport
  Pitch angle (deg) : Inport  Port=2
  Wind speed (m/s) : Inport  Port=3
  ->pu : Gain  Gain=1/Prated
  2-D Lookup Table1 : Lookup_n-D  BreakpointsForDimension1=breakpoints1  BreakpointsForDimension2=breakpoints2  Table=cp_table_data  InternalRulePriority=Speed  RndMeth=Simplest  InputSameDT=on
  Avoid div. by zero : Saturate  UpperLimit=inf  LowerLimit=eps
  "Avoid div. by zero " : Saturate  UpperLimit=inf  LowerLimit=eps
  Fcn1 : Fcn  Expr=K1*u[2]/u[1]
  Fcn2 : Fcn  Commented=on  Expr=c1*(c6*u[1] + (-c4 - c3*(2.5 + u[2]) + c2*(1/(u[1] + c7*(2.5 + u[2])) -c8/(1 + (2.5 + u[2])^3)))/exp(c5*(1/(u[1] + c7*(2.5 + u[2])) - c8/(1 + (2.5 + u[2])^3))))
  "K2*Cp*wind^3 " : Fcn  Expr=K2*u[1]^3*u[2]
  Mux : Mux  Inputs=2
  Mux2 : Mux  Inputs=2
  Product2 : Product  Inputs=*/  InputSameDT=on  SaturateOnIntegerOverflow=on  OutDataTypeStr=Inherit: Same as first input
  Tt (pu) : Outport  VectorParamsAs1DForOutWhenUnconnected=off
  wires:
  "K2*Cp*wind^3 "/1 -> ->pu/1
  "Avoid div. by zero "/1 -> Product2/2, Mux/2
  Avoid div. by zero/1 -> Mux/1, Mux2/1
  W_wt (pu)/1 -> "Avoid div. by zero "/1
  Pitch angle (deg)/1 -> 2-D Lookup Table1/2
  Mux2/1 -> "K2*Cp*wind^3 "/1
  2-D Lookup Table1/1 -> Mux2/2  "Cp"
  Mux/1 -> Fcn1/1
  Fcn1/1 -> 2-D Lookup Table1/1  "lambda"
  Wind speed (m/s)/1 -> Avoid div. by zero/1
  Product2/1 -> Tt (pu)/1
  ->pu/1 -> Product2/1  "power_pu"

== system Microgrid_transition_model_FORFIG/synchronous/EXCITATION ==
  Vref : Inport
  Vt : Inport  Port=2
  It : Inport  Port=3
  Ifd : Inport  Port=4
  Vstab : Inport  Port=5
  AC1A : Subsystem  VariantControl=Variant1
  AC4A : Subsystem  VariantControl=Variant2
  AC5A : Subsystem  VariantControl=Variant3
  DC1A : Subsystem  VariantControl=Variant4
  DC2A : Subsystem  VariantControl=Variant5
  ST1A : Subsystem  VariantControl=Variant6
  ST2A : sps_avr/ST2A Excitation System  VariantControl=Variant7  Tr=20e-3  KaTa=[120 0.15]  VRminmax=[0 1.0]  KfTf=[0.05 1.0]  KeTe=[1.0 0.5]  KI=8.0  Kp=4.88  Xd=1.56  Kc=1.82  v0=[1,1.42734]  I0=0.2739  TsBlock=-2
      settings: SourceProductBaseCode=PS
  Efd : Outport  VectorParamsAs1DForOutWhenUnconnected=off

== system Microgrid_transition_model_FORFIG/../Control/Excitation Control system ==
  Flux : Inport
  wr : Inport  Port=2
  Discrete PI Controller : Subsystem  DialogController=POWERSYS.PowerSysDialog  mask(Discrete PI Controller){Kp=Kp_field, Ki=Ki_field, Par_Limits=[1 0]*Vf_limit, Init=init(9), Ts=Ts}
      mask prompts: Kp "Proportional gain (Kp):"; Ki "Integral gain (Ki):"; Par_Limits "Output limits: [ Upper   Lower ]"; Init "Output initial value:"; Ts "Sample time:"
      mask help: This block implements a discrete PI controller.
      mask init:
      | UpperLimit=Par_Limits(1);
      | LowerLimit=Par_Limits(2);
      | power_initmask();
      mask Help: This block is part of a subset of blocks in the Extras library that does not have documentation associated with it, other than the block mask description.
      mask Display: disp('PI');
  Divide : Product  Inputs=*/
  Flux_ref : Constant
  "Flux_ref " : Constant
  Sum4 : Sum  Inputs=|+-  InputSameDT=on  SaturateOnIntegerOverflow=on  OutDataTypeStr=Inherit: Same as first input
  Switch : Switch  Threshold=1
  avoid division by 0 : Saturate  UpperLimit=inf  LowerLimit=1e-6
  Vf : Outport  VectorParamsAs1DForOutWhenUnconnected=off
  wires:
  Switch/1 -> Sum4/1
  Divide/1 -> Switch/1
  avoid division by 0/1 -> Divide/2
  "Flux_ref "/1 -> Divide/1
  Flux_ref/1 -> Switch/3
  wr/1 -> avoid division by 0/1, Switch/2
  Flux/1 -> Sum4/2  "Flux"
  Discrete PI Controller/1(Out) -> Vf/1  "Vf"
  Sum4/1 -> Discrete PI Controller/1(Error)

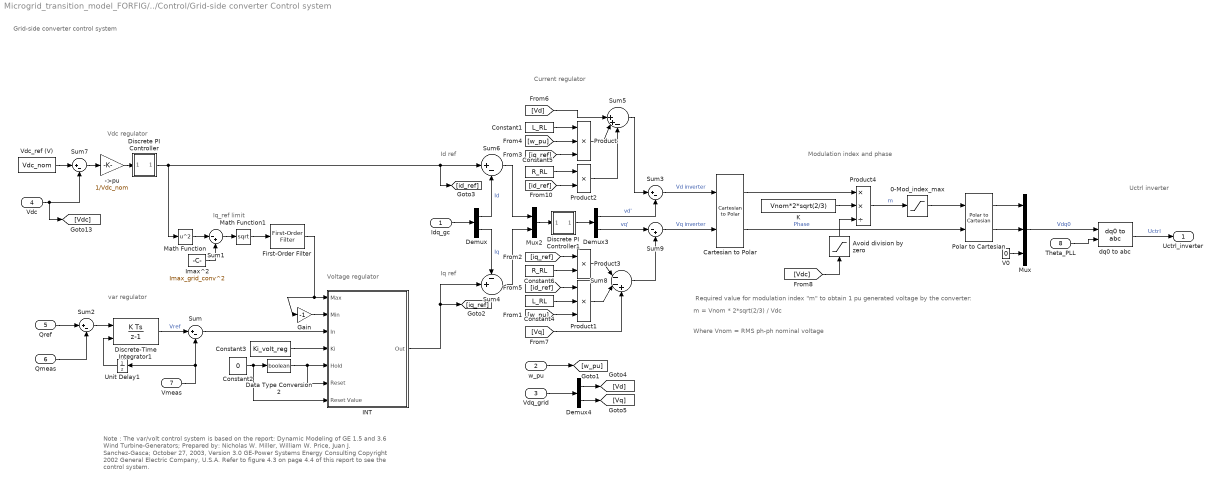
== system Microgrid_transition_model_FORFIG/../Control/Grid-side converter Control system ==
  note: Note :
      | The var/volt control system is based on the report:
      | Dynamic Modeling of GE 1.5 and 3.6 Wind Turbine-Generators;
      | Prepared by: Nicholas W. Miller, William W. Price, Juan J. Sanchez-Gasca;
      | October 27, 2003, Version 3.0
      | GE-Power Systems Energy Consulting
      | Copyright 2002 General Electric Company, U.S.A.
      |
      | Refer to figure 4.3 on page 4.4 of this report to see the control system.
  note: Uctrl inverter
  note: Modulation index and phase
  note: Where Vnom = RMS ph-ph nominal voltage
  note: m = Vnom * 2*sqrt(2/3) / Vdc
  note: Required value for modulation index "m" to obtain 1 pu generated voltage by the converter:
  note: Iq ref
  note: Id ref
  note: Current regulator
  note: Iq_ref limit
  note: Vdc regulator
  note: Voltage regulator
  note: var regulator
  note: Grid-side converter control system
  Idq_gc : Inport
  w_pu : Inport  Port=2
  Vdq_grid : Inport  Port=3
  Vdc : Inport  Port=4
  Qref : Inport  Port=5
  Qmeas : Inport  Port=6
  Vmeas : Inport  Port=7
  Theta_PLL : Inport  Port=8
  ->pu : Gain  Gain=1/Vdc_nom
  0-Mod_index_max : Saturate  UpperLimit=Mod_index_max  LowerLimit=0
  Avoid division by zero : Saturate  UpperLimit=1e6  LowerLimit=1e-6
  Cartesian to Polar : simulink_extras/Transformations/Cartesian to Polar
  Constant1 : Constant  Value=L_RL
  Constant2 : Constant  Value=0
  Constant3 : Constant  Value=Ki_volt_reg
  Constant4 : Constant  Value=L_RL
  Constant5 : Constant  Value=R_RL
  Constant6 : Constant  Value=R_RL
  Data Type Conversion2 : DataTypeConversion  OutDataTypeStr=boolean
  Demux : Demux  Outputs=2
      settings: DisplayOption=none
  Demux3 : Demux  Outputs=2
      settings: DisplayOption=none
  Demux4 : Demux  Outputs=2
      settings: DisplayOption=none
  Discrete PI Controller : Subsystem  DialogController=POWERSYS.PowerSysDialog  mask(Discrete PI Controller){Kp=Kp_dc, Ki=Ki_dc, Par_Limits=[1 -1]*Imax_grid_conv, Init=0, Ts=Ts}
      mask prompts: Kp "Proportional gain (Kp):"; Ki "Integral gain (Ki):"; Par_Limits "Output limits: [ Upper   Lower ]"; Init "Output initial value:"; Ts "Sample time:"
      mask help: This block implements a discrete PI controller.
      mask init:
      | UpperLimit=Par_Limits(1);
      | LowerLimit=Par_Limits(2);
      | power_initmask();
      mask Help: This block is part of a subset of blocks in the Extras library that does not have documentation associated with it, other than the block mask description.
      mask Display: disp('PI');
  Discrete PI Controller1 : Subsystem  DialogController=POWERSYS.PowerSysDialog  mask(Discrete PI Controller){Kp=Kp_grid_side_cur_reg, Ki=Ki_grid_side_cur_reg, Par_Limits=[1 -1]*Current_reg_output_limit, Init=0, Ts=Ts}
      mask prompts: Kp "Proportional gain (Kp):"; Ki "Integral gain (Ki):"; Par_Limits "Output limits: [ Upper   Lower ]"; Init "Output initial value:"; Ts "Sample time:"
      mask help: This block implements a discrete PI controller.
      mask init:
      | UpperLimit=Par_Limits(1);
      | LowerLimit=Par_Limits(2);
      | power_initmask();
      mask Help: This block is part of a subset of blocks in the Extras library that does not have documentation associated with it, other than the block mask description.
      mask Display: disp('PI');
  Discrete-Time Integrator1 : DiscreteIntegrator  gainval=Ki_var_reg  InitialConditionSource=external  InitialCondition=1  SampleTime=Ts  LimitOutput=on  UpperSaturationLimit=Var_reg_output_hi_limit  LowerSaturationLimit=Var_reg_output_low_limit  ICPrevOutput=DiscIntNeverNeededParam  ICPrevScaledInput=DiscIntNeverNeededParam
  First-Order Filter : powerlib_meascontrol/Filters/First-Order Filter  FilterType=Lowpass  Tc=Iq_ref_limit_time_constant  Ts=Ts  Initialize=on  Vac_Init=[0, 0, 0]  Vdc_Init=Imax_grid_conv  PlotResponse=off  FreqRange="[0,  200,  1]"
      settings: SourceProductBaseCode=MT,PS
  Gain : Gain  Gain=-1  SaturateOnIntegerOverflow=on  OutDataTypeStr=Inherit: Same as input  ParamDataTypeStr=Inherit: Same as input
  INT : Subsystem  mask(Integrator  With  External  Dynamic  Limits (Discrete)){}
      mask Display: disp('Discrete-Time\n(Trapezoidal)\nIntegrator\n ')
  Imax^2 : Constant  Value=Imax_grid_conv^2
  K : Constant  Value=Vnom*2*sqrt(2/3)
  Math Function : Math  Operator=square  SignedPower=on  SaturateOnIntegerOverflow=on
  Math Function1 : Math  Operator=sqrt  SignedPower=on  SaturateOnIntegerOverflow=on
  Mux : Mux  Inputs=3
  Mux2 : Mux  Inputs=2
  Polar to Cartesian : simulink_extras/Transformations/Polar to Cartesian
      settings: SourceProductBaseCode=SL
  Product : Product  Inputs=3  InputSameDT=on  SaturateOnIntegerOverflow=on  OutDataTypeStr=Inherit: Same as first input
  Product1 : Product  Inputs=3  InputSameDT=on  SaturateOnIntegerOverflow=on  OutDataTypeStr=Inherit: Same as first input
  Product2 : Product  InputSameDT=on  SaturateOnIntegerOverflow=on  OutDataTypeStr=Inherit: Same as first input
  Product3 : Product  InputSameDT=on  SaturateOnIntegerOverflow=on  OutDataTypeStr=Inherit: Same as first input
  Product4 : Product  Inputs=**/  InputSameDT=on  SaturateOnIntegerOverflow=on  OutDataTypeStr=Inherit: Same as first input
  Sum{,2..3,6..7} (5 alike) : Sum  Inputs=|+-  InputSameDT=on  SaturateOnIntegerOverflow=on  OutDataTypeStr=Inherit: Same as first input
  Sum1 : Sum  Inputs=|-+  InputSameDT=on  SaturateOnIntegerOverflow=on  OutDataTypeStr=Inherit: Same as first input
  Sum4 : Sum  Inputs=-+|  InputSameDT=on  SaturateOnIntegerOverflow=on  OutDataTypeStr=Inherit: Same as first input
  Sum5 : Sum  Inputs=||++-  InputSameDT=on  SaturateOnIntegerOverflow=on  OutDataTypeStr=Inherit: Same as first input
  Sum8 : Sum  Inputs=|--+  InputSameDT=on  SaturateOnIntegerOverflow=on  OutDataTypeStr=Inherit: Same as first input
  Sum9 : Sum  Inputs=|-+  InputSameDT=on  SaturateOnIntegerOverflow=on  OutDataTypeStr=Inherit: Same as first input
  Unit Delay1 : UnitDelay  InitialCondition=1  SampleTime=Ts  HasFrameUpgradeWarning=on
  V0 : Constant  Value=0
  Vdc_ref (V) : Constant  Value=Vdc_nom
  dq0 to abc : powerlib_meascontrol/Transformations/dq0 to abc  Alignment=90 degrees behind phase A axis
      settings: SourceProductBaseCode=MT,PS
  Uctrl_inverter : Outport  VectorParamsAs1DForOutWhenUnconnected=off
  wires:
  Theta_PLL/1 -> dq0 to abc/2
  INT/1(Out) -> [iq_ref], Sum4/2
  Qref/1 -> Sum2/1
  Vdc_ref (V)/1 -> Sum7/1
  Sum8/1 -> Sum9/2
  Sum5/1 -> Sum3/1
  0-Mod_index_max/1 -> Polar to Cartesian/1
  Idq_gc/1 -> Demux/1
  dq0 to abc/1 -> Uctrl_inverter/1  "Uctrl"
  Mux/1 -> dq0 to abc/1  "Vdq0"
  Cartesian to Polar/2 -> Polar to Cartesian/2  "Phase"
  V0/1 -> Mux/3
  Polar to Cartesian/1 -> Mux/1
  Polar to Cartesian/2 -> Mux/2
  Sum9/1 -> Cartesian to Polar/2  "Vq inverter"
  Sum3/1 -> Cartesian to Polar/1  "Vd inverter"
  [Vdc] -> Avoid division by zero/1
  Cartesian to Polar/1 -> Product4/1
  Avoid division by zero/1 -> Product4/3
  K/1 -> Product4/2
  Product4/1 -> 0-Mod_index_max/1  "m"
  [Vd] -> Sum5/1
  [Vq] -> Sum8/3
  Demux4/2 -> [Vq]
  Demux4/1 -> [Vd]
  w_pu/1 -> [w_pu]
  Demux3/2 -> Sum9/1  "vq'"
  Demux3/1 -> Sum3/2  "vd'"
  [id_ref] -> Product1/1
  [iq_ref] -> Product3/1
  [id_ref] -> Product2/2
  [iq_ref] -> Product/3
  [w_pu] -> Product/2
  [w_pu] -> Product1/3
  Sum4/1 -> Mux2/2
  Sum6/1 -> Mux2/1
  Product3/1 -> Sum8/1
  Product2/1 -> Sum5/3
  Product1/1 -> Sum8/2
  Constant6/1 -> Product3/2
  Constant5/1 -> Product2/1
  Product/1 -> Sum5/2
  Demux/1 -> Sum6/2  "Id"
  Demux/2 -> Sum4/1  "Iq"
  Constant1/1 -> Product/1
  Mux2/1 -> Discrete PI Controller1/1(Error)
  Discrete PI Controller1/1(Out) -> Demux3/1
  Constant4/1 -> Product1/2
  First-Order Filter/1 -> INT/1(Max), Gain/1
  Math Function/1 -> Sum1/1
  Imax^2/1 -> Sum1/2
  Sum1/1 -> Math Function1/1
  Math Function1/1 -> First-Order Filter/1
  Unit Delay1/1 -> Discrete-Time Integrator1/2
  Sum2/1 -> Discrete-Time Integrator1/1
  Qmeas/1 -> Sum2/2
  Vmeas/1 -> Sum/2, Unit Delay1/1
  Discrete-Time Integrator1/1 -> Sum/1  "Vref"
  Constant3/1 -> INT/4(Ki)
  Gain/1 -> INT/2(Min)
  Data Type Conversion2/1 -> INT/6(Reset), INT/5(Hold)
  Constant2/1 -> INT/7(Reset Value), Data Type Conversion2/1
  Sum/1 -> INT/3(In)
  Discrete PI Controller/1(Out) -> Sum6/1, [id_ref], Math Function/1
  ->pu/1 -> Discrete PI Controller/1(Error)
  Sum7/1 -> ->pu/1
  Vdq_grid/1 -> Demux4/1
  Vdc/1 -> Sum7/2, [Vdc]
